simulink model "firstOrderSim"  (R2013a)
settings: Solver=ode45  StartTime=0.0  StopTime=787  RelTol=1e-3
values from neighbouring files (symbols this model uses):
  gain = delta_y/delta_x    [findGain.m]    (also in firstOrder.m = findGain(A, B, init_offset, final_offset, sample_size))
undefined symbols (not defined in the file or in its folder): init_diff, init_time, time
settings Model: Creator=root  LastModifiedBy=root

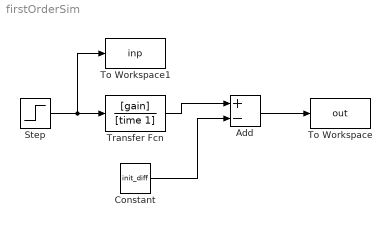
== system firstOrderSim ==
  Add : Sum  Inputs=+-
  Constant : Constant  Value=init_diff
  Step : Step  Time=init_time/10  After=2  SampleTime=0
  To Workspace : ToWorkspace  VariableName=out  SampleTime=-1  SaveFormat=Timeseries
  To Workspace1 : ToWorkspace  VariableName=inp  SampleTime=-1  SaveFormat=Timeseries
  Transfer Fcn : TransferFcn  Numerator=[gain]  Denominator=[time 1]
  wires:
  Step/1 -> To Workspace1/1, Transfer Fcn/1
  Constant/1 -> Add/2
  Transfer Fcn/1 -> Add/1
  Add/1 -> To Workspace/1
